simulink model "imc"  (R2021a)
settings: Solver=VariableStepAuto  StartTime=0.0  StopTime=250  RelTol=1e-3
values from neighbouring files (symbols this model uses):
  K = b(end) / (1-exp(-Ts/T))    [Workflow.m]
  T = -Ts/log(abs(a(end)))    [Workflow.m]
  T_process = T    [Workflow.m]
  T_regulation = 15    [Workflow.m]
  Ts = 1    [Workflow.m]    (also in main.m = 0.01)
undefined symbols (not defined in the file or in its folder): D
libraries: simulink x1
settings Model: Creator=VY259YA  LastModifiedBy=VY259YA

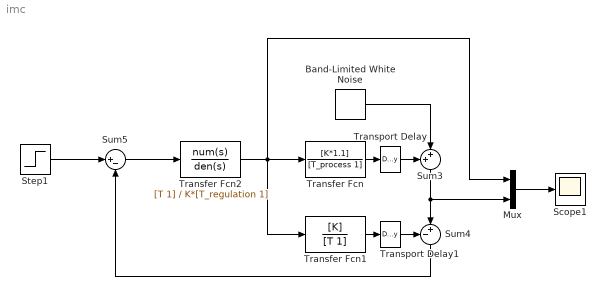
== system imc ==
  Band-Limited White Noise : simulink/Sources/Band-Limited White Noise  Cov=[0.001]  Ts=0.1  seed=[23341]
  Mux : Mux  Inputs=2
  Scope1 : Scope
  Step1 : Step  Time=0  SampleTime=Ts
  Sum3 : Sum  Inputs=++|
  Sum4 : Sum  Inputs=-+|
  Sum5 : Sum  Inputs=|+-
  Transfer Fcn : TransferFcn  Numerator=[K*1.1]  Denominator=[T_process 1]
  Transfer Fcn1 : TransferFcn  Numerator=[K]  Denominator=[T 1]
  Transfer Fcn2 : TransferFcn  Numerator=[T 1]  Denominator=K*[T_regulation 1]
  Transport Delay : TransportDelay  DelayTime=D
  Transport Delay1 : TransportDelay  DelayTime=D
  wires:
  Transfer Fcn2/1 -> Transfer Fcn1/1, Mux/1, Transfer Fcn/1
  Sum3/1 -> Mux/2, Sum4/2
  Transfer Fcn1/1 -> Transport Delay1/1
  Transfer Fcn/1 -> Transport Delay/1
  Step1/1 -> Sum5/1
  Sum5/1 -> Transfer Fcn2/1
  Sum4/1 -> Sum5/2
  Mux/1 -> Scope1/1
  Band-Limited White Noise/1 -> Sum3/2
  Transport Delay/1 -> Sum3/1
  Transport Delay1/1 -> Sum4/1
